simulink model "HOG"  (R2022a)
settings: Solver=VariableStepAuto  StartTime=0.0  StopTime=15  RelTol=1e-3
model workspace (MATLAB code in the model file):
  | P1 = [2 0.5 1.6];
  | P2 = [2 -0.5 1.6];
  | P3 = [1.6 0.5 0.9];
  | P4 = [1.6 0 0.9];
  | P5 = [2 0.5 1.6];
  | 
  | t_sim = [0 10];
  | 
  | BlueBase_L = 0.8;
  | BlueBrick_L = 0.3;
  | Red_L = 1.05;
  | Green_L = 0.8;
  | GreenBrick_L = 0.3;
  | White_L = 1.05;
  | LBlue_L = 0.4;
  | Grey_L = 1.175;
  | Black_L = 0.2;
undefined symbols (not defined in the file): B, Spline, X, Y, Z
libraries: sm_lib x47, nesl_utility x12, robotcorelib x3
(part 2 of 2)

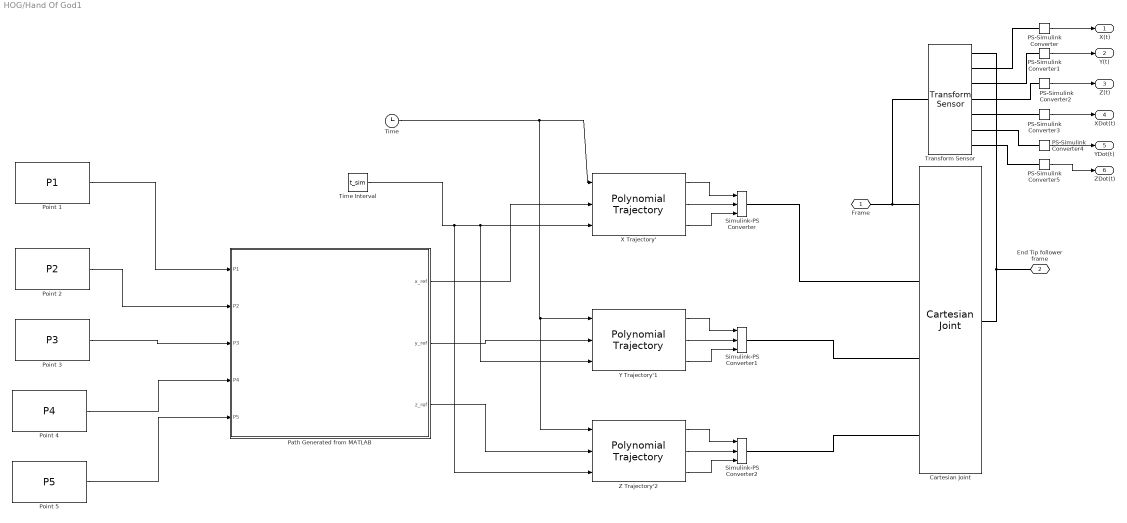
== system HOG/Hand Of God1 ==
  Cartesian Joint : sm_lib/Joints/Cartesian Joint  JointMode=Normal  SenseConstraintForce=off  SenseConstraintForceX=off  SenseConstraintForceY=off  SenseConstraintForceZ=off  SenseConstraintTorque=off  SenseConstraintTorqueX=off  SenseConstraintTorqueY=off  SenseConstraintTorqueZ=off  SenseTotalForce=off  SenseTotalForceX=off  SenseTotalForceY=off  SenseTotalForceZ=off  SenseTotalTorque=off  SenseTotalTorqueX=off  SenseTotalTorqueY=off  SenseTotalTorqueZ=off  CompositeWrenchDir=FollowerOnBase  CompositeWrenchFrame=BaseFrame  PxEquilibriumPosition=0  PxEquilibriumPositionUnits=m  PxSpringStiffness=0  PxSpringStiffnessUnits=N/m  PxDampingCoefficient=0  PxDampingCoefficientUnits=N/(m/s)  PxTorqueActuationMode=ComputedTorque  PxMotionActuationMode=InputMotion  PxSensePosition=off  PxSenseVelocity=off  PxSenseAcceleration=off  PxSenseTorqueForce=off  PxSenseLowerLimitTorqueForce=off  PxSenseUpperLimitTorqueForce=off  PxLowerLimitSpecify=off  PxLowerLimitBound=-1  PxLowerLimitBoundUnits=m  PxLowerLimitStiffness=1e6  PxLowerLimitStiffnessUnits=N/m  PxLowerLimitDamping=1e3  PxLowerLimitDampingUnits=N/(m/s)  PxLowerLimitTransitionRegionWidth=1e-4  PxLowerLimitTransitionRegionWidthUnits=m  PxUpperLimitSpecify=off  PxUpperLimitBound=1  PxUpperLimitBoundUnits=m  PxUpperLimitStiffness=1e6  PxUpperLimitStiffnessUnits=N/m  PxUpperLimitDamping=1e3  PxUpperLimitDampingUnits=N/(m/s)  PxUpperLimitTransitionRegionWidth=1e-4  PxUpperLimitTransitionRegionWidthUnits=m  PxPositionTargetSpecify=off  PxPositionTargetPriority=High  PxPositionTargetValue=0  PxPositionTargetValueUnits=m  PxVelocityTargetSpecify=off  PxVelocityTargetPriority=High  PxVelocityTargetValue=0  PxVelocityTargetValueUnits=m/s  PyEquilibriumPosition=0  PyEquilibriumPositionUnits=m  PySpringStiffness=0  PySpringStiffnessUnits=N/m  PyDampingCoefficient=0  PyDampingCoefficientUnits=N/(m/s)  PyTorqueActuationMode=ComputedTorque  PyMotionActuationMode=InputMotion  PySensePosition=off  PySenseVelocity=off  PySenseAcceleration=off  PySenseTorqueForce=off  PySenseLowerLimitTorqueForce=off  PySenseUpperLimitTorqueForce=off  PyLowerLimitSpecify=off  PyLowerLimitBound=-1  PyLowerLimitBoundUnits=m  PyLowerLimitStiffness=1e6  PyLowerLimitStiffnessUnits=N/m  PyLowerLimitDamping=1e3  PyLowerLimitDampingUnits=N/(m/s)  PyLowerLimitTransitionRegionWidth=1e-4  PyLowerLimitTransitionRegionWidthUnits=m  PyUpperLimitSpecify=off  PyUpperLimitBound=1  PyUpperLimitBoundUnits=m  PyUpperLimitStiffness=1e6  PyUpperLimitStiffnessUnits=N/m  PyUpperLimitDamping=1e3  PyUpperLimitDampingUnits=N/(m/s)  PyUpperLimitTransitionRegionWidth=1e-4  PyUpperLimitTransitionRegionWidthUnits=m  PyPositionTargetSpecify=off  PyPositionTargetPriority=High  PyPositionTargetValue=0  PyPositionTargetValueUnits=m  PyVelocityTargetSpecify=off  PyVelocityTargetPriority=High  PyVelocityTargetValue=0  PyVelocityTargetValueUnits=m/s  PzEquilibriumPosition=0  PzEquilibriumPositionUnits=m  PzSpringStiffness=0  PzSpringStiffnessUnits=N/m  PzDampingCoefficient=0  PzDampingCoefficientUnits=N/(m/s)  PzTorqueActuationMode=ComputedTorque  PzMotionActuationMode=InputMotion  PzSensePosition=off  PzSenseVelocity=off  PzSenseAcceleration=off  PzSenseTorqueForce=off  PzSenseLowerLimitTorqueForce=off  PzSenseUpperLimitTorqueForce=off  PzLowerLimitSpecify=off  PzLowerLimitBound=-1  PzLowerLimitBoundUnits=m  PzLowerLimitStiffness=1e6  PzLowerLimitStiffnessUnits=N/m  PzLowerLimitDamping=1e3  PzLowerLimitDampingUnits=N/(m/s)  PzLowerLimitTransitionRegionWidth=1e-4  PzLowerLimitTransitionRegionWidthUnits=m  PzUpperLimitSpecify=off  PzUpperLimitBound=1  PzUpperLimitBoundUnits=m  PzUpperLimitStiffness=1e6  PzUpperLimitStiffnessUnits=N/m  PzUpperLimitDamping=1e3  PzUpperLimitDampingUnits=N/(m/s)  PzUpperLimitTransitionRegionWidth=1e-4  PzUpperLimitTransitionRegionWidthUnits=m  PzPositionTargetSpecify=off  PzPositionTargetPriority=High  PzPositionTargetValue=0  PzPositionTargetValueUnits=m  PzVelocityTargetSpecify=off  PzVelocityTargetPriority=High  PzVelocityTargetValue=0  PzVelocityTargetValueUnits=m/s
  PS-Simulink Converter{,1..5} (6 alike) : nesl_utility/PS-Simulink Converter  PhysicalDomain=network_engine_domain  SubClassName=ps_output  LeftPortType=input  RightPortType=output  PseudoPeriodic=off  Frequencies=[]  VectorFormat=inherit  Unit=inherit  AffineConversion=off
      settings: SourceProductBaseCode=SS,PW,VE
  Path Generated from MATLAB : MATLAB Function  TreatAsAtomicUnit=on
  Point 1 : Constant  Value=P1
  Point 2 : Constant  Value=P2
  Point 3 : Constant  Value=P3
  Point 4 : Constant  Value=P4
  Point 5 : Constant  Value=P5
  Simulink-PS Converter : nesl_utility/Simulink-PS Converter  PhysicalDomain=network_engine_domain  SubClassName=ps_input  LeftPortType=input  RightPortType=output  PseudoPeriodic=off  Frequencies=[]  NoiseDistribution=none  NoiseParameters=[]  Unit=1  AffineConversion=off  FilteringAndDerivatives=provide  SimscapeFilterOrder=1  InputFilterTimeConstant=0.001  UdotUserProvided=2
      settings: SourceProductBaseCode=SS,PW,VE
  Simulink-PS Converter1 : nesl_utility/Simulink-PS Converter  PhysicalDomain=network_engine_domain  SubClassName=ps_input  LeftPortType=input  RightPortType=output  PseudoPeriodic=off  Frequencies=[]  NoiseDistribution=none  NoiseParameters=[]  Unit=1  AffineConversion=off  FilteringAndDerivatives=provide  SimscapeFilterOrder=1  InputFilterTimeConstant=0.001  UdotUserProvided=2
      settings: SourceProductBaseCode=SS,PW,VE
  Simulink-PS Converter2 : nesl_utility/Simulink-PS Converter  PhysicalDomain=network_engine_domain  SubClassName=ps_input  LeftPortType=input  RightPortType=output  PseudoPeriodic=off  Frequencies=[]  NoiseDistribution=none  NoiseParameters=[]  Unit=1  AffineConversion=off  FilteringAndDerivatives=provide  SimscapeFilterOrder=1  InputFilterTimeConstant=0.001  UdotUserProvided=2
      settings: SourceProductBaseCode=SS,PW,VE
  Time : Clock
  Time Interval : Constant  Value=t_sim
  Transform Sensor : sm_lib/Frames and Transforms/Transform Sensor  MeasurementFrame=World  SenseAngle=off  SenseAxis=off  SenseAngle1=off  SenseAngle2=off  SenseAngle3=off  SenseQ=off  SenseR=off  SenseOmegaX=off  SenseOmegaY=off  SenseOmegaZ=off  SenseOmega1=off  SenseOmega2=off  SenseOmega3=off  SenseQDot=off  SenseRDot=off  SenseAlphaX=off  SenseAlphaY=off  SenseAlphaZ=off  SenseAlpha1=off  SenseAlpha2=off  SenseAlpha3=off  SenseQDDot=off  SenseRDDot=off  SenseX=on  SenseY=on  SenseZ=on  SenseRad=off  SenseAzim=off  SenseDist=off  SenseInc=off  SenseXDot=on  SenseYDot=on  SenseZDot=on  SenseRadDot=off  SenseAzimDot=off  SenseDistDot=off  SenseIncDot=off  SenseXDDot=off  SenseYDDot=off  SenseZDDot=off  SenseRadDDot=off  SenseAzimDDot=off  SenseDistDDot=off  SenseIncDDot=off
  X Trajectory' : robotcorelib/Polynomial Trajectory  WaypointSource=External  Waypoints=[ 0, 2, 1, 5, 0; -1, 3, 1, 4, 4 ]  TimePoints=[ 0, 1, 2, 3, 4 ]  TimeInterval=[ 1, 4 ]  Method=B-Spline  ParameterSource=Internal  VelocityBoundaryCondition=zeros( 2, 5 )  AccelerationBoundaryCondition=zeros( 2, 5 )  SimulateUsing=Interpreted execution
      settings: SourceProductBaseCode=RO,NV,RR,UV
  Y Trajectory'1 : robotcorelib/Polynomial Trajectory  WaypointSource=External  Waypoints=[ 0, 2, 1, 5, 0; -1, 3, 1, 4, 4 ]  TimePoints=[ 0, 1, 2, 3, 4 ]  TimeInterval=[ 1, 4 ]  Method=B-Spline  ParameterSource=Internal  VelocityBoundaryCondition=zeros( 2, 5 )  AccelerationBoundaryCondition=zeros( 2, 5 )  SimulateUsing=Interpreted execution
      settings: SourceProductBaseCode=RO,NV,RR,UV
  Z Trajectory'2 : robotcorelib/Polynomial Trajectory  WaypointSource=External  Waypoints=[ 0, 2, 1, 5, 0; -1, 3, 1, 4, 4 ]  TimePoints=[ 0, 1, 2, 3, 4 ]  TimeInterval=[ 1, 4 ]  Method=B-Spline  ParameterSource=Internal  VelocityBoundaryCondition=zeros( 2, 5 )  AccelerationBoundaryCondition=zeros( 2, 5 )  SimulateUsing=Interpreted execution
      settings: SourceProductBaseCode=RO,NV,RR,UV
  Frame : PMIOPort  Side=Left
  End Tip follower frame : PMIOPort  Port=2  Side=Right
  X(t) : Outport
  Y(t) : Outport  Port=2
  Z(t) : Outport  Port=3
  XDot(t) : Outport  Port=4
  YDot(t) : Outport  Port=5
  ZDot(t) : Outport  Port=6
  wires:
  Point 1/1 -> Path Generated from MATLAB/1(P1)
  Point 2/1 -> Path Generated from MATLAB/2(P2)
  Point 3/1 -> Path Generated from MATLAB/3(P3)
  Point 4/1 -> Path Generated from MATLAB/4(P4)
  Point 5/1 -> Path Generated from MATLAB/5(P5)
  Path Generated from MATLAB/1(x_ref) -> X Trajectory'/2
  Time/1 -> Z Trajectory'2/1, Y Trajectory'1/1, X Trajectory'/1
  Path Generated from MATLAB/2(y_ref) -> Y Trajectory'1/2
  Path Generated from MATLAB/3(z_ref) -> Z Trajectory'2/2
  Time Interval/1 -> Z Trajectory'2/3, Y Trajectory'1/3, X Trajectory'/3
  X Trajectory'/1 -> Simulink-PS Converter/1
  X Trajectory'/2 -> Simulink-PS Converter/2
  X Trajectory'/3 -> Simulink-PS Converter/3
  Y Trajectory'1/3 -> Simulink-PS Converter1/3
  Y Trajectory'1/1 -> Simulink-PS Converter1/1
  Y Trajectory'1/2 -> Simulink-PS Converter1/2
  Z Trajectory'2/3 -> Simulink-PS Converter2/3
  Z Trajectory'2/1 -> Simulink-PS Converter2/1
  Z Trajectory'2/2 -> Simulink-PS Converter2/2
  PS-Simulink Converter/1 -> X(t)/1
  PS-Simulink Converter2/1 -> Z(t)/1
  PS-Simulink Converter1/1 -> Y(t)/1
  PS-Simulink Converter3/1 -> XDot(t)/1
  PS-Simulink Converter4/1 -> YDot(t)/1
  PS-Simulink Converter5/1 -> ZDot(t)/1
  connections:
  Frame/RConn1 -- Transform Sensor/LConn1 -- Cartesian Joint/LConn1
  Simulink-PS Converter/RConn1 -- Cartesian Joint/LConn2
  Simulink-PS Converter1/RConn1 -- Cartesian Joint/LConn3
  Simulink-PS Converter2/RConn1 -- Cartesian Joint/LConn4
  Cartesian Joint/RConn1 -- End Tip follower frame/RConn1 -- Transform Sensor/RConn1
  PS-Simulink Converter/LConn1 -- Transform Sensor/RConn2
  Transform Sensor/RConn3 -- PS-Simulink Converter1/LConn1
  Transform Sensor/RConn4 -- PS-Simulink Converter2/LConn1
  PS-Simulink Converter3/LConn1 -- Transform Sensor/RConn5
  PS-Simulink Converter4/LConn1 -- Transform Sensor/RConn6
  PS-Simulink Converter5/LConn1 -- Transform Sensor/RConn7

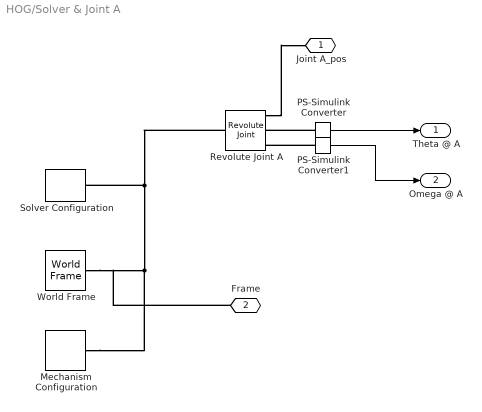
== system HOG/Solver & Joint A ==
  Mechanism Configuration : sm_lib/Utilities/Mechanism Configuration  UniformGravity=Constant  GravityVector=[0 0 -9.80665]  GravityUnits=m/s^2  LinearizationDelta=0.001  JointModeTransitionNonlinearIterations=2
  PS-Simulink Converter : nesl_utility/PS-Simulink Converter  PhysicalDomain=network_engine_domain  SubClassName=ps_output  LeftPortType=input  RightPortType=output  PseudoPeriodic=off  Frequencies=[]  VectorFormat=inherit  Unit=inherit  AffineConversion=off
      settings: SourceProductBaseCode=SS,PW,VE
  PS-Simulink Converter1 : nesl_utility/PS-Simulink Converter  PhysicalDomain=network_engine_domain  SubClassName=ps_output  LeftPortType=input  RightPortType=output  PseudoPeriodic=off  Frequencies=[]  VectorFormat=inherit  Unit=inherit  AffineConversion=off
      settings: SourceProductBaseCode=SS,PW,VE
  Revolute Joint A : sm_lib/Joints/Revolute Joint  JointMode=Normal  SenseConstraintForce=off  SenseConstraintForceX=off  SenseConstraintForceY=off  SenseConstraintForceZ=off  SenseConstraintTorque=off  SenseConstraintTorqueX=off  SenseConstraintTorqueY=off  SenseConstraintTorqueZ=off  SenseTotalForce=off  SenseTotalForceX=off  SenseTotalForceY=off  SenseTotalForceZ=off  SenseTotalTorque=off  SenseTotalTorqueX=off  SenseTotalTorqueY=off  SenseTotalTorqueZ=off  CompositeWrenchDir=FollowerOnBase  CompositeWrenchFrame=BaseFrame  EquilibriumPosition=0  EquilibriumPositionUnits=deg  SpringStiffness=0  SpringStiffnessUnits=N*m/deg  DampingCoefficient=0  DampingCoefficientUnits=N*m/(deg/s)  TorqueActuationMode=NoTorque  MotionActuationMode=ComputedMotion  SensePosition=on  SenseVelocity=on  SenseAcceleration=off  SenseTorqueForce=off  SenseLowerLimitTorqueForce=off  SenseUpperLimitTorqueForce=off  LowerLimitSpecify=off  LowerLimitBound=-90  LowerLimitBoundUnits=deg  LowerLimitStiffness=1e4  LowerLimitStiffnessUnits=N*m/deg  LowerLimitDamping=10  LowerLimitDampingUnits=N*m/(deg/s)  LowerLimitTransitionRegionWidth=0.1  LowerLimitTransitionRegionWidthUnits=deg  UpperLimitSpecify=off  UpperLimitBound=90  UpperLimitBoundUnits=deg  UpperLimitStiffness=1e4  UpperLimitStiffnessUnits=N*m/deg  UpperLimitDamping=10  UpperLimitDampingUnits=N*m/(deg/s)  UpperLimitTransitionRegionWidth=0.1  UpperLimitTransitionRegionWidthUnits=deg  PositionTargetSpecify=off  PositionTargetPriority=High  PositionTargetValue=0  PositionTargetValueUnits=deg  VelocityTargetSpecify=off  VelocityTargetPriority=High  VelocityTargetValue=0  VelocityTargetValueUnits=deg/s
  Solver Configuration : nesl_utility/Solver Configuration  PhysicalDomain=network_engine_domain  SubClassName=solver  LeftPortType=input  RightPortType=generic  Tones=[]  Harmonics=[]  SimulateNoise=off  Profile=off  UseLocalSampling=off  EnableSwitchedLinearOptims=on  FrequencyDomain=off  UseCCode=off  RelTol=0.001  AbsTol=1e-06  MinStep=1e-09  ToWorkspace=off  RevertToSquareIcSolve=off  NumHomotopyIterations=100  PhasorMode=off  PhasorModeNumHarmonics=1  IndexReductionMethod=DerivativeReplacement  DoDC=off  ResidualTolerance=1e-09  UseLocalSolver=off  LocalSolverChoice=NE_BACKWARD_EULER_ADVANCER  LocalSolverSampleTime=0.001  DoFixedCost=off  MaxNonlinIter=3  MaxModeIter=2  ComputeImpulses=off  ImpulseIterations=2  LinearAlgebra=Sparse  LinearAlgebraNumThread=0  EquationFormulation=NE_TIME_EF  DelaysMemoryBudget=1024  AutomaticFiltering=on  FilteringTimeConstant=0.001  PartitionStorageMethod=AS_NEEDED  PartitionMemoryBudget=1024  PartitionMethod=FAST
      settings: SourceProductBaseCode=SS,PW,VE
  World Frame : sm_lib/Frames and Transforms/World Frame
  Joint A_pos : PMIOPort  Side=Right
  Frame : PMIOPort  Port=2  Side=Right
  Theta @ A : Outport
  Omega @ A : Outport  Port=2
  wires:
  PS-Simulink Converter/1 -> Theta @ A/1
  PS-Simulink Converter1/1 -> Omega @ A/1
  connections:
  Revolute Joint A/LConn1 -- Solver Configuration/RConn1 -- Frame/RConn1 -- World Frame/RConn1 -- Mechanism Configuration/RConn1
  Revolute Joint A/RConn1 -- Joint A_pos/RConn1
  PS-Simulink Converter/LConn1 -- Revolute Joint A/RConn2
  PS-Simulink Converter1/LConn1 -- Revolute Joint A/RConn3

== matlab function HOG/Hand Of God1/Path Generated from MATLAB ==
  data: x_ref output; y_ref output; P1 input; P2 input; P3 input; P4 input; P5 input; z_ref output
function [x_ref, y_ref, z_ref] = fcn(P1, P2, P3, P4, P5)


%Position, velocity and acceleration
%P1
x1 = 2; %meters
x1Dot = 0.0; % No velocity
x1DotDot = 0.0; % No acceleration -> robot is stationary in rest position

y1 = 0.5;
y1Dot = 0.0;
y1DotDot = 0.0;

z1 = 1.6;
z1Dot = 0.0;
z1DotDot = 0.0;

%P2
x2 = 2;
x2Dot = -0.3;
x2DotDot = -0.1; 

y2 = -0.5;
y2Dot = -0.2;
y2DotDot = -0.05; 

z2 = 1.6;
z2Dot = -0.1;
z2DotDot = -0.05; 

%P3
x3 = 1.6;
x3Dot = -0.3;
x3DotDot = -0.05;

y3 = 0.5;
y3Dot = -0.2;
y3DotDot = -0.05; 

z3 = 0.9;
z3Dot = -0.2;
z3DotDot = -0.02;

% P4
x4 = 1.6;
x4Dot = 0.2;
x4DotDot = 0.1;

y4 = 0;
y4Dot = 0.2;
y4DotDot = 0.1;

z4 = 0.9;
z4Dot = 0.3;
z4DotDot = 0.1;

%P5
x5 = 2; 
x5Dot = 0.0;
x5DotDot = 0.0;

y5 = 0.5;
y5Dot = 0.0;
y5DotDot = 0.0;

z5 = 1.6;
z5Dot = 0.0;
z5DotDot = 0.0; 

%Arbitary Constants (Timestamps for each point, t1, t2...)
T1 = 0;
T2 = 1;
T3 = 2;
T4 = 3;
T5 = 4; 

%Timeintervals for the piecewise curve fitting
dt = 0.01;

t1 = [T1:dt:T2];
t2 = [T2:dt:T3]; 
t3 = [T3:dt:T4]; 
t4 = [T4:dt:T5]; 

%Column vectors for the position, velocity and acceleration for each point
%including arbitary constants. Arbitary constants indicate position and
%velocity at the endpoint of each curve, i.e. position and velocity at the
%next point. For the last point, acceleration must also be included to make
%the robot stop as accurately as possible. 

%P1(t1) -> P1(t2)
X1 = [x1; x1Dot; x1DotDot; x2; x2Dot];
Y1 = [y1; y1Dot; y1DotDot; y2; y2Dot]; 
Z1 = [z1; z1Dot; z1DotDot; z2; z2Dot]; 

%P2(t2) -> P2(t3)
X2 = [x2; x2Dot; x2DotDot; x3; x3Dot];
Y2 = [y2; y2Dot; y2DotDot; y3; y3Dot]; 
Z2 = [z2; z2Dot; z2DotDot; z3; z3Dot];

%P3(t3) -> P3(t4)
X3 = [x3; x3Dot; x3DotDot; x4; x4Dot];
Y3 = [y3; y3Dot; y3DotDot; y4; y4Dot]; 
Z3 = [z3; z3Dot; z3DotDot; z4; z4Dot];

%P4(t4) -> P4(t5)
X4 = [x4; x4Dot; x4DotDot; x5; x5Dot; x5DotDot];
Y4 = [y4; y4Dot; y4DotDot; y5; y5Dot; y5DotDot]; 
Z4 = [z4; z4Dot; z4DotDot; z5; z5Dot; z5DotDot];

%Adding the matrices including the polynomials for each curve w/ its
%derivatives
  
A_1 = [F3(T1); F3Dot(T1); F3DotDot(T1); F3(T2); F3Dot(T2)]; 
A_2 = [F3(T2); F3Dot(T2); F3DotDot(T2); F3(T3); F3Dot(T3)];
A_3 = [F3(T3); F3Dot(T3); F3DotDot(T3); F3(T4); F3Dot(T4)]; 
A_4 = [F4(T4); F4Dot(T4); F4DotDot(T4); F4(T5); F4Dot(T5); F4DotDot(T5)]; 
   
% Finding matrices of the unknowns for each point

AX1 = (A_1)\X1; 
AY1 = (A_1)\Y1;
AZ1 = (A_1)\Z1; 

BX2 = (A_2)\X2;
BY2 = (A_2)\Y2;
BZ2 = (A_2)\Z2;

CX3 = (A_3)\X3;
CY3 = (A_3)\Y3;
CZ3 = A_3\Z3;

DX4 = (A_4)\X4;
DY4 = (A_4)\Y4;
DZ4 = (A_4)\Z4; 

% Setting up the polynomial equations for each point in XYZ
%P1 at t = t1 
X_p1 = F(t1, AX1); 
Y_p1 = F(t1, AY1);
Z_p1 = F(t1, AZ1); 

%P2 at t = t2
X_p2 = F(t2, BX2);
Y_p2 = F(t2, BY2);
Z_p2 = F(t2, BZ2); 

% P3 at t = t3
X_p3 = F(t3, CX3);
Y_p3 = F(t3, CY3);
Z_p3 = F(t3, CZ3); 

% P4 at t = t4
X_p4 = F1(t4, DX4);
Y_p4 = F1(t4, DY4);
Z_p4 = F1(t4, DZ4); 

X_Out = [X_p1 X_p2 X_p3 X_p4];
Y_Out = [Y_p1 Y_p2 Y_p3 Y_p4];
Z_Out = [Z_p1 Z_p2 Z_p3 Z_p4]; 

x_ref = X_Out;
y_ref = Y_Out;
z_ref = Z_Out; 


function[out] = F(t, b)
out = [ b(1) + b(2)*t + b(3)*t.^2 + b(4)*t.^3 + b(5)*t.^4];
end 

function[out] = F1(t, b)
out = [ b(1) + b(2)*t + b(3)*t.^2 + b(4)*t.^3 + b(5)*t.^4 + b(6)*t.^5];
end

function [out] = F4(t) 
out =   [1   t    t.^2    t.^3     t.^4   t.^5];
end

function [out] = F4Dot(t)
out =   [0   1    2*t    3*t.^2   4*t.^3  5*t^4];
end

function [out] = F4DotDot(t)
out = [0   0   2   6*t    12*t.^2    20*t^3];
end

function [out] = F3(t) 
out =   [1   t    t.^2    t.^3   t.^4];
end

function [out] = F3Dot(t)
out =   [0   1    2*t    3*t.^2   4*t.^3];
end

function [out] = F3DotDot(t)
out = [0   0    2    6*t   12*t.^2];
end
end
